simulink model "SAD_project_full_mission"  (R2023b)
settings: Solver=ode4  StartTime=0.0  StopTime=tf  FixedStep=t_step  RelTol=1e-3
values from neighbouring files (symbols this model uses):
  A1 = importdata("igrfSg.txt")    [SAD_project_code.m]
  A2 = importdata("igrfSh.txt")    [SAD_project_code.m]
  A_1 = area_face(1)    [SAD_project_code.m]
  A_2 = area_face(2)    [SAD_project_code.m]
  A_3 = area_face(3)    [SAD_project_code.m]
  A_4 = area_face(4)    [SAD_project_code.m]
  A_5 = area_face(5)    [SAD_project_code.m]
  A_6 = area_face(6)    [SAD_project_code.m]
  alpha = [1/1000 99/1000]    [SAD_project_code.m]
  DCM_eci_per = rotationMatrix(rad2deg(i),rad2deg(OM), rad2deg(om))    [SAD_project_code.m]
  e = 0.0011241    [SAD_project_code.m]
  FS = 50000e-9    (= 5e-05)    [SAD_project_code.m]
  H0 = [g_10 g_11 h_11]'    [SAD_project_code.m]
  h_r_0 = [0,0,0]'    [SAD_project_code.m]
  horizon_cone_limit = deg2rad(359)    [SAD_project_code.m]
  I = 5/12.*diag([Ix Iy Iz])    [SAD_project_code.m]
  i = deg2rad(97.55)    [SAD_project_code.m]
  I_inv = inv(I)    [SAD_project_code.m]
  I_RW = 3.32e-3    (= 0.00332)    [SAD_project_code.m]
  I_vector_RW = [I_RW I_RW I_RW]'    [SAD_project_code.m]
  inc_tot = sqrt(inc_lin^2 + inc_acc^2)    [SAD_project_code.m]
  InitialTrueAnomalyOfEarth = 0    [SAD_project_code.m]
  j_b = [0.001 0.005 0.001]'    [SAD_project_code.m]
  K1_point = lqr(A, B, Q, R)    [SAD_project_code.m]
  K1_slew = 0.8    [SAD_project_code.m]
  K2_point = K1_point.^2/2    [SAD_project_code.m]
  K2_slew = K1_slew.^2/2    [SAD_project_code.m]
  K_detumbling = lqr(A,B,Q,R)    [SAD_project_code.m]
  matrix_RW_config = eye(3)    [SAD_project_code.m]
  matrix_RW_config_inv = inv(matrix_RW_config)    [SAD_project_code.m]
  mu_E = astroConstants(13)    [SAD_project_code.m]
  N_1 = BODY(1,:)    [SAD_project_code.m]
  N_2 = BODY(2,:)    [SAD_project_code.m]
  N_3 = BODY(3,:)    [SAD_project_code.m]
  N_4 = BODY(4,:)    [SAD_project_code.m]
  N_5 = BODY(5,:)    [SAD_project_code.m]
  N_6 = BODY(6,:)    [SAD_project_code.m]
  n_earth = sqrt(mu_E/a^3)    [SAD_project_code.m]
  om = deg2rad(206.3209)    [SAD_project_code.m]
  OM = deg2rad(50.7464)    [SAD_project_code.m]
  p = a*(1-e^2)    [SAD_project_code.m]
  q0 = q0/norm(q0)    [SAD_project_code.m]
  r_1 = r(1,:)    [SAD_project_code.m]
  r_2 = r(2,:)    [SAD_project_code.m]
  r_3 = r(3,:)    [SAD_project_code.m]
  r_4 = r(4,:)    [SAD_project_code.m]
  r_5 = r(5,:)    [SAD_project_code.m]
  r_6 = r(6,:)    [SAD_project_code.m]
  R_E = astroConstants(23)    [SAD_project_code.m]
  rho_d1 = 0.1    [SAD_project_code.m]
  rho_d2 = 0.1    [SAD_project_code.m]
  rho_d3 = 0.1    [SAD_project_code.m]
  rho_d4 = 0.1    [SAD_project_code.m]
  rho_d5 = 0.1    [SAD_project_code.m]
  rho_d6 = 0.1    [SAD_project_code.m]
  rho_s1 = rho_s(1)    [SAD_project_code.m]
  rho_s2 = rho_s(2)    [SAD_project_code.m]
  rho_s3 = rho_s(3)    [SAD_project_code.m]
  rho_s4 = rho_s(4)    [SAD_project_code.m]
  rho_s5 = rho_s(5)    [SAD_project_code.m]
  rho_s6 = rho_s(6)    [SAD_project_code.m]
  t_step = 0.1    [SAD_project_code.m]
  th0 = deg2rad(0)    [SAD_project_code.m]
  timeoflaunch = date2mjd2000(date0)    [SAD_project_code.m]
  torque_max = 47.1e-3    (= 0.0471)    [SAD_project_code.m]
  ts_sensor = 5*t_step    (= 0.05)    [SAD_project_code.m]
  w0 = rand(3,1)    [SAD_project_code.m]
  w0_RW = [0 0 0]    [SAD_project_code.m]
  w_E = deg2rad(15.04)/60/60    [SAD_project_code.m]
  wMax_RW = 2*pi * RPM_max_RW / 60    (= 680.678408278)    [SAD_project_code.m]
libraries: matrix_library x28, sharedtransform x5, simulink_extras x4, simulink x3, dspindex x3, vrlib x2, dspinverses x1, aerolibutil x1
(part 1 of 4)
settings Model: Creator=samue  LastModifiedBy=samue

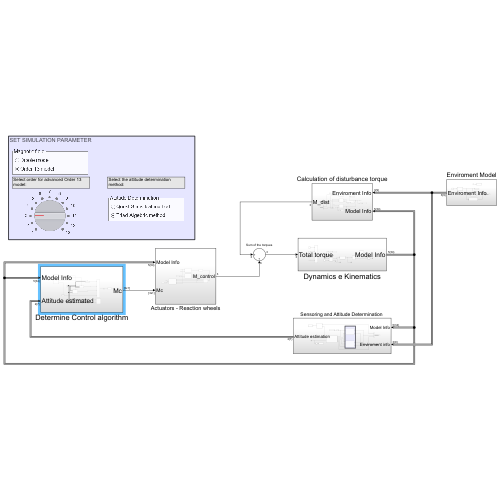
[thumbnail: Simulink's stored preview of the top-level diagram]
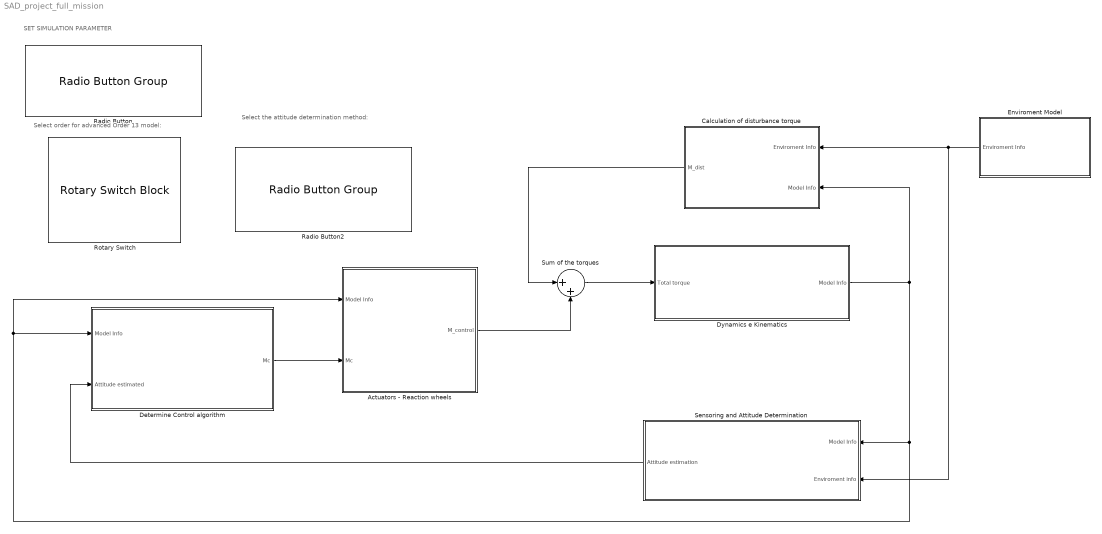
== system SAD_project_full_mission ==
  note: Select the attitude determination method:
  note: SET SIMULATION PARAMETER
  note: Select order for advanced Order 13 model:
  Actuators - Reaction wheels : Subsystem
  Calculation of disturbance torque : Subsystem
  Determine Control algorithm : Subsystem
  Dynamics e Kinematics : Subsystem
  Enviroment Model : Subsystem
  Radio Button : RadioButtonGroup  LabelPosition=Hide  SelectedLabel=Order 13 model  ButtonGroupName=Magnetic field
      settings: Values={{'Dipole model', 'Order 13 model'}, [0 1]}
  Radio Button2 : RadioButtonGroup  LabelPosition=Hide  SelectedLabel=Triad-Algebric method  ButtonGroupName=Attitude Determination
      settings: Values={{'Quest-Statisitcal method', 'Triad-Algebric method'}, [1 2]}
  Rotary Switch : RotarySwitchBlock  LabelPosition=Hide
      settings: Values={{'1', '2', '3', '4', '5', '6', '7', '8', '9', '10', '11', '12', '13'}, [1 2 3 4 5 6 7 8 9 10 11 12 13]}
  "Sensoring and Attitude Determination " : Subsystem
  Sum of the torques : Sum  Inputs=|++
  wires:
  Sum of the torques/1 -> Dynamics e Kinematics/1(Total torque)
  Actuators - Reaction wheels/1(M_control) -> Sum of the torques/2
  Enviroment Model/1(Enviroment Info) -> "Sensoring and Attitude Determination "/2(Enviroment info), Calculation of disturbance torque/1(Enviroment Info)
  Dynamics e Kinematics/1(Model Info) -> Actuators - Reaction wheels/1(Model Info), Determine Control algorithm/1(Model Info), "Sensoring and Attitude Determination "/1(Model Info), Calculation of disturbance torque/2(Model Info)
  "Sensoring and Attitude Determination "/1(Attitude estimation) -> Determine Control algorithm/2(Attitude estimated)
  Calculation of disturbance torque/1(M_dist) -> Sum of the torques/1
  Determine Control algorithm/1(Mc) -> Actuators - Reaction wheels/2(Mc)

== system SAD_project_full_mission/Actuators - Reaction wheels ==
  BusElementIn : Inport  PortName=Model Info  Element=w_b true
  Mc : Inport  Port=2
  Calculatate wRW in base of saturation : Subsystem
  Integration on omega RW : Subsystem
  Reaction wheel model : Subsystem
  Reshape : Reshape
  Reshape4 : Reshape
  Subsystem1 : Subsystem
  To Workspace1 : ToWorkspace  VariableName=wr  SampleTime=-1
  To Workspace6 : ToWorkspace  VariableName=M_actuator  SampleTime=-1
  detect if the RW is saturated (output == 1 isSaturated) : Subsystem
  M_control : Outport
  wires:
  detect if the RW is saturated (output == 1 isSaturated)/2(flag RW2) -> Calculatate wRW in base of saturation/3(flag RW2 (1 is saturated)), Subsystem1/2(flag RW2 (1 is saturated))  "flag RW2 (1 is saturated)"
  Calculatate wRW in base of saturation/1(wRW) -> Reshape/1
  Mc/1 -> Subsystem1/4(Mc), Reaction wheel model/1(Mc)
  detect if the RW is saturated (output == 1 isSaturated)/3(flag RW3) -> Calculatate wRW in base of saturation/4(flag RW3 (1 is saturated)), Subsystem1/3(flag RW3 (1 is saturated))  "flag RW3 (1 is saturated)"
  detect if the RW is saturated (output == 1 isSaturated)/1(flag RW1) -> Calculatate wRW in base of saturation/2(flag RW1 (1 is saturated)), Subsystem1/1(flag RW1 (1 is saturated))  "flag RW1 (1 is saturated)"
  Reshape/1 -> To Workspace1/1
  Subsystem1/1(M) -> M_control/1, Reshape4/1
  Reshape4/1 -> To Workspace6/1
  BusElementIn/1 -> Reaction wheel model/2(w_b true)
  Reaction wheel model/1(h_r dot) -> Integration on omega RW/1(In1)
  Integration on omega RW/1(wRW integrated) -> Calculatate wRW in base of saturation/1(wRW integrated), detect if the RW is saturated (output == 1 isSaturated)/1(w)

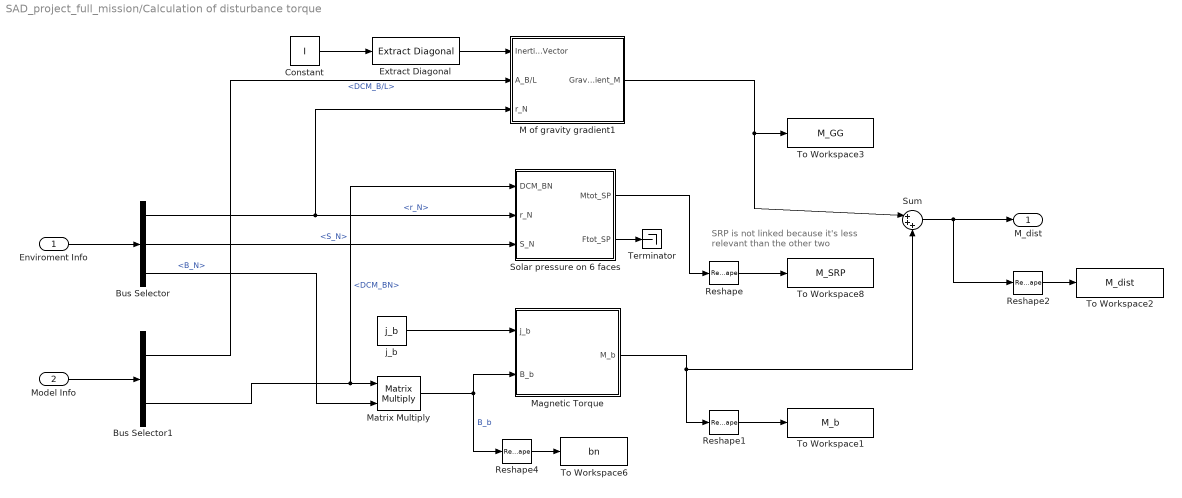
== system SAD_project_full_mission/Calculation of disturbance torque ==
  note: SRP is not linked because it's less relevant than the other two
  Enviroment Info : Inport
  Model Info : Inport  Port=2
  Bus Selector : BusSelector  OutputSignals=r_N,S_N,B_N
  Bus Selector1 : BusSelector  OutputSignals=DCM_B/L,DCM_BN
  Constant : Constant  Value=I
  Extract Diagonal : matrix_library/Extract Diagonal
      settings: LibrarySourceBlock=|
      | simulink/Matrix
      | Operations/Extract Diagonal
  M of gravity gradient1 : Subsystem
  Magnetic Torque : Subsystem
  Matrix Multiply : Product  Multiplication=Matrix(*)
  Reshape{,1..2,4} (4 alike) : Reshape
  Solar pressure on 6 faces : Subsystem
  Sum : Sum  Inputs=|+++
  Terminator : Terminator
  To Workspace1 : ToWorkspace  VariableName=M_b  SampleTime=-1
  To Workspace2 : ToWorkspace  VariableName=M_dist  SampleTime=-1
  To Workspace3 : ToWorkspace  VariableName=M_GG  SampleTime=-1
  To Workspace6 : ToWorkspace  VariableName=bn  SampleTime=-1
  To Workspace8 : ToWorkspace  VariableName=M_SRP  SampleTime=-1
  j_b : Constant  Value=j_b
  M_dist : Outport
  wires:
  j_b/1 -> Magnetic Torque/1(j_b)
  Magnetic Torque/1(M_b) -> Sum/3, Reshape1/1
  Sum/1 -> Reshape2/1, M_dist/1
  Reshape/1 -> To Workspace8/1
  Reshape1/1 -> To Workspace1/1
  M of gravity gradient1/1(GravityGradient_M) -> Sum/1, To Workspace3/1
  Solar pressure on 6 faces/2(Ftot_SP) -> Terminator/1
  Solar pressure on 6 faces/1(Mtot_SP) -> Reshape/1
  Extract Diagonal/1 -> M of gravity gradient1/1(Inertia Vector)
  Reshape4/1 -> To Workspace6/1
  Matrix Multiply/1 -> Reshape4/1, Magnetic Torque/2(B_b)  "B_b"
  Enviroment Info/1 -> Bus Selector/1
  Constant/1 -> Extract Diagonal/1
  Bus Selector/1 -> M of gravity gradient1/3(r_N), Solar pressure on 6 faces/2("r_N ")  "<r_N>"
  Bus Selector/2 -> Solar pressure on 6 faces/3(S_N)  "<S_N>"
  Model Info/1 -> Bus Selector1/1
  Bus Selector1/1 -> M of gravity gradient1/2(A_B/L)  "<DCM_B/L>"
  Reshape2/1 -> To Workspace2/1
  Bus Selector/3 -> Matrix Multiply/2  "<B_N>"
  Bus Selector1/2 -> Solar pressure on 6 faces/1(DCM_BN), Matrix Multiply/1  "<DCM_BN>"

== system SAD_project_full_mission/Determine Control algorithm ==
  Model Info : Inport
  Attitude estimated : Inport  Port=2
  Bus Selector : BusSelector  OutputSignals=q estimated
  Bus Selector1 : BusSelector  OutputSignals=A_L/N
  Check if the Mc is finite : Subsystem
  Clock : Clock
  DCM to quaternion : Subsystem
  If : If  IfExpression=u1 > 500  ElseIfExpressions=u1 > 350, u1 > 120
  Merge : Merge  Inputs=4
  "Saturation +- Max RW torque " : Saturate  UpperLimit=torque_max  LowerLimit=-torque_max
  Switch Case Action 3 axis stabilization Algorithm : Subsystem  TreatAsAtomicUnit=on
  Switch Case Action Detumle Algorithm : Subsystem  TreatAsAtomicUnit=on
  Switch Case Action Mc = 0 : Subsystem  TreatAsAtomicUnit=on
  Switch Case Action Slew Maneuver Algorithm : Subsystem  TreatAsAtomicUnit=on
  To Workspace data : Subsystem
  Mc : Outport
  wires:
  Switch Case Action Slew Maneuver Algorithm/1(Mc) -> Merge/2
  Switch Case Action Detumle Algorithm/1(Mc) -> Merge/1
  Switch Case Action 3 axis stabilization Algorithm/1(Mc) -> Merge/3
  Merge/1 -> "Saturation +- Max RW torque "/1  "Control Moment"
  Attitude estimated/1 -> Switch Case Action Slew Maneuver Algorithm/2(Attitude estimated), Switch Case Action Detumle Algorithm/1(Attitude estimated), Switch Case Action 3 axis stabilization Algorithm/2(Attitude estimated), Bus Selector/1
  Clock/1 -> If/1
  Model Info/1 -> Bus Selector1/1, Switch Case Action Slew Maneuver Algorithm/1(Model info), Switch Case Action 3 axis stabilization Algorithm/1(Model info)
  Switch Case Action Mc = 0/1(Output) -> Merge/4
  Bus Selector/1 -> To Workspace data/2(<q estimated>)  "<q estimated>"
  If/4 -> Switch Case Action Mc = 0/Action  "No control"
  If/1 -> Switch Case Action 3 axis stabilization Algorithm/Action  "3 axis Stabilisation"
  If/2 -> Switch Case Action Slew Maneuver Algorithm/Action  "Slew Maneuver"
  If/3 -> Switch Case Action Detumle Algorithm/Action  "Detumble case"
  "Saturation +- Max RW torque "/1 -> Check if the Mc is finite/1(Mc)
  Check if the Mc is finite/1(Control Moment) -> Mc/1
  Bus Selector1/1 -> DCM to quaternion/1(DCM)  "<A_L/N>"
  DCM to quaternion/1(q (scalar last)) -> To Workspace data/1(q target)

== system SAD_project_full_mission/Dynamics e Kinematics ==
  Total torque : Inport
  Constant6 : Constant  Value=q0
  DCM composition from quaternions 1 : Subsystem  AncestorBlock=LibrarySAD5/DCM composition from quaternions
  From A_B/N to A_B/L and A_L/N : Subsystem
  Inertia Matrix : Constant  Value=I  VectorParams1D=off
  "Initial ω " : Constant  Value=w0
  Inverse Inertia Matrix : Constant  Value=I_inv
  Kinematics with quaternions : Subsystem
  Matrix Multiply : Product  Multiplication=Matrix(*)
  Real Omega : ToWorkspace  VariableName=w  SampleTime=-1
  Reshape1 : Reshape
  Rotation of -90 degree around y axis : Constant  Value=[0 0 -1; 0 1 0; 1 0 0]
  Single spin dynamics : Subsystem  AncestorBlock=My_library/Single spin dynamics
  Terminator1 : Terminator
  Transpose : Math  Operator=transpose
  Out Bus Element : Outport  PortName=Model Info  Element=w_b true
  Out Bus Element2 : Outport  PortName=Model Info  Element=DCM_B/L
  Out Bus Element3 : Outport  PortName=Model Info  Element=q_b True
  Out Bus Element4 : Outport  PortName=Model Info  Element=DCM_BN
  Out Bus Element5 : Outport  PortName=Model Info  Element=A_L/N
  wires:
  Single spin dynamics/1(Omega) -> Kinematics with quaternions/1(omega), Transpose/1, Reshape1/1  "real ω_B"
  Total torque/1 -> Single spin dynamics/4(M)
  Inverse Inertia Matrix/1 -> Single spin dynamics/1(Inertia matrix inverse)
  Inertia Matrix/1 -> Single spin dynamics/2(Inertia matrix)
  "Initial ω "/1 -> Single spin dynamics/3(Omega_0)
  Constant6/1 -> Kinematics with quaternions/2(q0)
  Kinematics with quaternions/1(q) -> Out Bus Element3/1, DCM composition from quaternions 1/1(q(4x1))  "q_b True"
  Reshape1/1 -> Real Omega/1
  Kinematics with quaternions/2(q^(-1)) -> Terminator1/1
  DCM composition from quaternions 1/1(DCM) -> Out Bus Element4/1, From A_B/N to A_B/L and A_L/N/1(DCM_B/N)  "DCM_BN"
  From A_B/N to A_B/L and A_L/N/1(DCM_B/L) -> Out Bus Element2/1
  Transpose/1 -> Out Bus Element/1
  Rotation of -90 degree around y axis/1 -> Matrix Multiply/1
  From A_B/N to A_B/L and A_L/N/2(A_L/N) -> Matrix Multiply/2
  Matrix Multiply/1 -> Out Bus Element5/1

== system SAD_project_full_mission/Enviroment Model ==
  Bus Creator : BusCreator  Inputs=3
  Clock : Clock
  Constant4 : Constant  Value=th0
  Magnetic Field : Subsystem
  Sun Position in Earth Centred Equatorial Inertial RF : Subsystem
  To Workspace : ToWorkspace  VariableName=r_N  SampleTime=-1
  To Workspace1 : ToWorkspace  VariableName=t  SampleTime=-1
  two-body Keplerian dynamics ECI : Subsystem
  Enviroment Info : Outport
  wires:
  Constant4/1 -> two-body Keplerian dynamics ECI/1(th0)
  Sun Position in Earth Centred Equatorial Inertial RF/1(s_N) -> Bus Creator/2  "S_N"
  two-body Keplerian dynamics ECI/1(r_N) -> Magnetic Field/1(r_N), Bus Creator/1, To Workspace/1  "r_N"
  Magnetic Field/1(B_N) -> Bus Creator/3  "B_N"
  Bus Creator/1 -> Enviroment Info/1
  Clock/1 -> To Workspace1/1

== system SAD_project_full_mission/Sensoring and Attitude Determination  ==
  note: error between the true q and the estimated one
  note: Sensors
  Model Info : Inport
  Enviroment info : Inport  Port=2
  Attitude Determination : Subsystem
  Bus Selector : BusSelector  OutputSignals=B_N,r_N
  Bus Selector1 : BusSelector  OutputSignals=q_b True,DCM_BN,w_b true
  Horizon Sensor : Subsystem
  MAG-3  Magnetometer1 : Subsystem
  Relative attitude error with quaternion : Subsystem
  Reshape : Reshape
  Reshape3 : Reshape
  To Workspace : ToWorkspace  VariableName=w_est  SampleTime=-1
  To Workspace1 : ToWorkspace  VariableName=q_error  SampleTime=-1
  To Workspace5 : ToWorkspace  VariableName=b_sensor  SampleTime=-1
  Out Bus Element2 : Outport  PortName=Attitude estimation  Element=q estimated
  Out Bus Element1 : Outport  PortName=Attitude estimation  Element=w estimated
  wires:
  MAG-3  Magnetometer1/2(B_n) -> Attitude Determination/2(B_N)
  Horizon Sensor/1(Perturbed data Horizon) -> Attitude Determination/3(Horizon_b sensor)  "R_b perturbed sensor"
  Horizon Sensor/2(R_N Horizon) -> Attitude Determination/4(Horizon_N)
  MAG-3  Magnetometer1/1(B_b perturbed sensor) -> Attitude Determination/1(B_b sensor), Reshape3/1
  Bus Selector/1 -> MAG-3  Magnetometer1/2(B_N)  "<B_N>"
  Enviroment info/1 -> Bus Selector/1
  Bus Selector/2 -> Horizon Sensor/2(R_N)  "<r_N>"
  Bus Selector1/2 -> Horizon Sensor/1(DCM_B/N), MAG-3  Magnetometer1/1(DCM_B/N)  "<DCM_BN>"
  Reshape3/1 -> To Workspace5/1
  Model Info/1 -> Bus Selector1/1
  Relative attitude error with quaternion/1(qe) -> To Workspace1/1
  Bus Selector1/1 -> Relative attitude error with quaternion/1(q_b true)  "<q_b True>"
  Attitude Determination/1(q estimated) -> Relative attitude error with quaternion/2(estimated q), Out Bus Element2/1
  Reshape/1 -> To Workspace/1
  Attitude Determination/2(w estimated) -> Reshape/1, Out Bus Element1/1
  Horizon Sensor/3(Flag If Earth is visible) -> Attitude Determination/5(Flag IsEarthVisible)
  Bus Selector1/3 -> Attitude Determination/6(Input)  "<w_b true>"

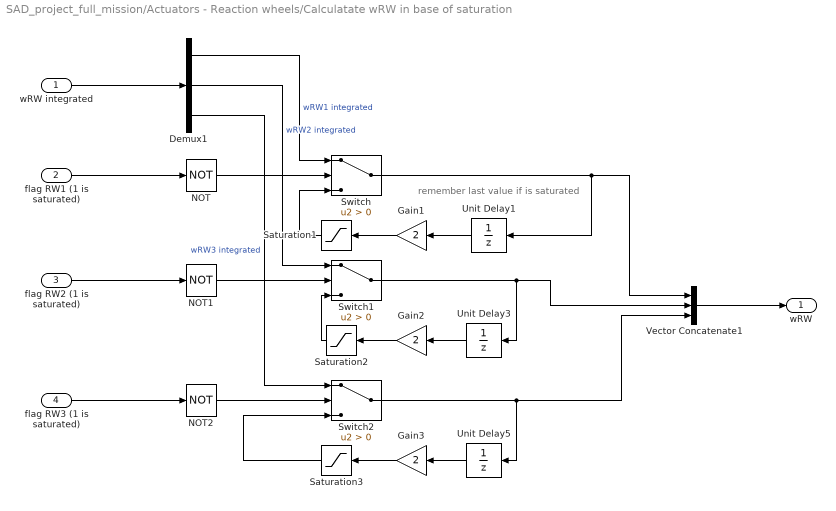
== system SAD_project_full_mission/Actuators - Reaction wheels/Calculatate wRW in base of saturation ==
  note: remember last value if is saturated
  wRW integrated : Inport
  flag RW1 (1 is saturated) : Inport  Port=2
  flag RW2 (1 is saturated) : Inport  Port=3
  flag RW3 (1 is saturated) : Inport  Port=4
  Demux1 : Demux  Outputs=3
  Gain1 : Gain  Gain=2
  Gain2 : Gain  Gain=2
  Gain3 : Gain  Gain=2
  NOT : Logic  Operator=NOT  IconShape=distinctive  AllPortsSameDT=off  OutDataTypeStr=boolean
  NOT1 : Logic  Operator=NOT  IconShape=distinctive  AllPortsSameDT=off  OutDataTypeStr=boolean
  NOT2 : Logic  Operator=NOT  IconShape=distinctive  AllPortsSameDT=off  OutDataTypeStr=boolean
  Saturation1 : Saturate  UpperLimit=wMax_RW  LowerLimit=-wMax_RW
  Saturation2 : Saturate  UpperLimit=wMax_RW  LowerLimit=-wMax_RW
  Saturation3 : Saturate  UpperLimit=wMax_RW  LowerLimit=-wMax_RW
  Switch : Switch  Criteria=u2 > Threshold  SaturateOnIntegerOverflow=off  InputSameDT=off
  Switch1 : Switch  Criteria=u2 > Threshold  SaturateOnIntegerOverflow=off  InputSameDT=off
  Switch2 : Switch  Criteria=u2 > Threshold  SaturateOnIntegerOverflow=off  InputSameDT=off
  Unit Delay1 : UnitDelay  SampleTime=-1  HasFrameUpgradeWarning=on
  Unit Delay3 : UnitDelay  SampleTime=-1  HasFrameUpgradeWarning=on
  Unit Delay5 : UnitDelay  SampleTime=-1  HasFrameUpgradeWarning=on
  Vector Concatenate1 : Concatenate  NumInputs=3
  wRW : Outport
  wires:
  Gain2/1 -> Saturation2/1
  Switch1/1 -> Unit Delay3/1, Vector Concatenate1/2
  NOT/1 -> Switch/2
  flag RW1 (1 is saturated)/1 -> NOT/1
  Saturation3/1 -> Switch2/3
  NOT1/1 -> Switch1/2
  Saturation2/1 -> Switch1/3
  wRW integrated/1 -> Demux1/1
  Switch2/1 -> Unit Delay5/1, Vector Concatenate1/3
  Unit Delay5/1 -> Gain3/1
  Unit Delay3/1 -> Gain2/1
  Demux1/2 -> Switch1/1  "wRW2 integrated"
  Gain1/1 -> Saturation1/1
  Vector Concatenate1/1 -> wRW/1
  Switch/1 -> Unit Delay1/1, Vector Concatenate1/1
  Unit Delay1/1 -> Gain1/1
  Saturation1/1 -> Switch/3
  Demux1/3 -> Switch2/1  "wRW3 integrated"
  Demux1/1 -> Switch/1  "wRW1 integrated"
  NOT2/1 -> Switch2/2
  Gain3/1 -> Saturation3/1
  flag RW3 (1 is saturated)/1 -> NOT2/1
  flag RW2 (1 is saturated)/1 -> NOT1/1

== system SAD_project_full_mission/Actuators - Reaction wheels/Integration on omega RW ==
  In1 : Inport
  Constant3 : Constant  Value=I_vector_RW
  Constant9 : Constant  Value=w0_RW
  Divide : Product  Inputs=*/
  Integrator1 : Integrator  InitialConditionSource=external
  wRW integrated : Outport
  wires:
  Divide/1 -> Integrator1/1  "wRW dot"
  Constant9/1 -> Integrator1/2
  Constant3/1 -> Divide/2
  Integrator1/1 -> wRW integrated/1  "wRW integrated"
  In1/1 -> Divide/1

== system SAD_project_full_mission/Actuators - Reaction wheels/Reaction wheel model ==
  Mc : Inport
  w_b true : Inport  Port=2
  Constant5 : Constant  Value=h_r_0  VectorParams1D=off
  Constant6 : Constant  Value=matrix_RW_config  VectorParams1D=off
  Constant8 : Constant  Value=matrix_RW_config_inv  VectorParams1D=off
  Cross Product : matrix_library/Cross Product
  Gain : Gain  Gain=-1
  Integrator : Integrator  InitialConditionSource=external
  Matrix Multiply : Product  Multiplication=Matrix(*)
  Matrix Multiply1 : Product  Multiplication=Matrix(*)
  Saturation : Saturate  UpperLimit=wMax_RW*I_RW  LowerLimit=-wMax_RW*I_RW
  Sum : Sum  Inputs=|++
  h_r dot : Outport
  wires:
  Constant5/1 -> Integrator/2
  Constant6/1 -> Matrix Multiply/1
  Sum/1 -> Matrix Multiply1/2
  Integrator/1 -> Saturation/1  "h_r"
  Matrix Multiply/1 -> Cross Product/2
  Constant8/1 -> Gain/1
  Cross Product/1 -> Sum/2
  Gain/1 -> Matrix Multiply1/1
  Matrix Multiply1/1 -> h_r dot/1, Integrator/1  "h_r dot"
  Saturation/1 -> Matrix Multiply/2
  Mc/1 -> Sum/1
  w_b true/1 -> Cross Product/1

== system SAD_project_full_mission/Actuators - Reaction wheels/Subsystem1 ==
  flag RW1 (1 is saturated) : Inport
  flag RW2 (1 is saturated) : Inport  Port=2
  flag RW3 (1 is saturated) : Inport  Port=3
  Mc : Inport  Port=4
  Band-Limited White Noise : simulink/Sources/Band-Limited White Noise  Cov=[0.00001, 0.00001, 0.00001]'  Ts=t_step  seed=[23341]
  Constant10 : Constant  Value=0
  Constant11 : Constant  Value=0
  Constant7 : Constant  Value=0
  Demux3 : Demux  Outputs=3
  Sum : Sum  Inputs=|++
  Switch1 : Switch  Criteria=u2 > Threshold  SaturateOnIntegerOverflow=off  InputSameDT=off
  Switch2 : Switch  Criteria=u2 > Threshold  SaturateOnIntegerOverflow=off  InputSameDT=off
  Switch3 : Switch  Criteria=u2 > Threshold  SaturateOnIntegerOverflow=off  InputSameDT=off
  Vector Concatenate2 : Concatenate  NumInputs=3
  M : Outport
  wires:
  Demux3/2 -> Switch1/3
  Constant11/1 -> Switch2/1
  Constant7/1 -> Switch3/1
  flag RW2 (1 is saturated)/1 -> Switch1/2
  flag RW1 (1 is saturated)/1 -> Switch3/2
  Demux3/3 -> Switch2/3
  Constant10/1 -> Switch1/1
  Demux3/1 -> Switch3/3
  flag RW3 (1 is saturated)/1 -> Switch2/2
  Switch3/1 -> Vector Concatenate2/1
  Switch1/1 -> Vector Concatenate2/2
  Switch2/1 -> Vector Concatenate2/3
  Vector Concatenate2/1 -> M/1
  Mc/1 -> Sum/1
  Sum/1 -> Demux3/1

== system SAD_project_full_mission/Actuators - Reaction wheels/detect if the RW is saturated (output == 1 isSaturated) ==
  w : Inport
  Abs : Abs  SaturateOnIntegerOverflow=off
  Compare To Constant : simulink/Logic and Bit Operations/Compare To Constant  relop=>=  const=wMax_RW  OutDataTypeStr=boolean
  Demux : Demux  Outputs=3
  Logical Operator : Logic  Operator=OR  AllPortsSameDT=off  OutDataTypeStr=boolean
  Logical Operator1 : Logic  Operator=OR  AllPortsSameDT=off  OutDataTypeStr=boolean
  Logical Operator2 : Logic  Operator=OR  AllPortsSameDT=off  OutDataTypeStr=boolean
  Unit Delay : UnitDelay  SampleTime=-1  HasFrameUpgradeWarning=on
  Unit Delay2 : UnitDelay  SampleTime=-1  HasFrameUpgradeWarning=on
  Unit Delay4 : UnitDelay  SampleTime=-1  HasFrameUpgradeWarning=on
  flag RW1 : Outport
  flag RW2 : Outport  Port=2
  flag RW3 : Outport  Port=3
  wires:
  Unit Delay4/1 -> Logical Operator2/2
  Unit Delay/1 -> Logical Operator/2
  Demux/1 -> Logical Operator/1
  Logical Operator/1 -> flag RW1/1, Unit Delay/1
  Unit Delay2/1 -> Logical Operator1/2
  Logical Operator2/1 -> flag RW3/1, Unit Delay4/1
  Demux/2 -> Logical Operator1/1
  Logical Operator1/1 -> flag RW2/1, Unit Delay2/1
  Demux/3 -> Logical Operator2/1
  Abs/1 -> Compare To Constant/1
  w/1 -> Abs/1
  Compare To Constant/1 -> Demux/1

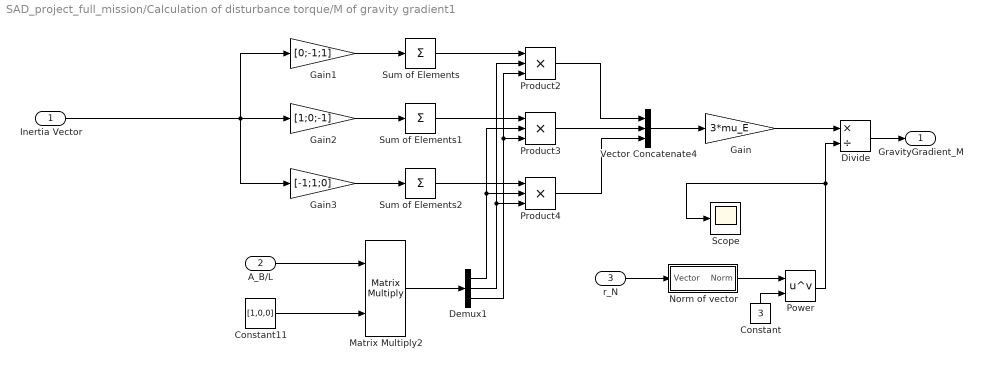
== system SAD_project_full_mission/Calculation of disturbance torque/M of gravity gradient1 ==
  Inertia Vector : Inport
  A_B/L : Inport  Port=2
  r_N : Inport  Port=3
  Constant : Constant  Value=3
  Constant11 : Constant  Value=[1,0,0]
  Demux1 : Demux  Outputs=3
  Divide : Product  Inputs=*/
  Gain : Gain  Gain=3*mu_E
  Gain1 : Gain  Gain=[0;-1;1]
  Gain2 : Gain  Gain=[1;0;-1]
  Gain3 : Gain  Gain=[-1;1;0]
  Matrix Multiply2 : Product  Multiplication=Matrix(*)
  Norm of vector : Subsystem  AncestorBlock=LibrarySAD5/Normalize Vector1
  Power : Math  Operator=pow
  Product2 : Product  Inputs=3
  Product3 : Product  Inputs=3
  Product4 : Product  Inputs=3
  Scope : Scope
  Sum of Elements : Sum  Inputs=+
  Sum of Elements1 : Sum  Inputs=+
  Sum of Elements2 : Sum  Inputs=+
  Vector Concatenate4 : Concatenate  NumInputs=3
  GravityGradient_M : Outport
  wires:
  Demux1/3 -> Product2/3, Product3/3
  Product2/1 -> Vector Concatenate4/1
  Matrix Multiply2/1 -> Demux1/1
  Product4/1 -> Vector Concatenate4/3
  Product3/1 -> Vector Concatenate4/2
  Demux1/1 -> Product4/2, Product3/2
  Constant11/1 -> Matrix Multiply2/2
  Demux1/2 -> Product4/3, Product2/2
  A_B/L/1 -> Matrix Multiply2/1
  Vector Concatenate4/1 -> Gain/1
  Gain1/1 -> Sum of Elements/1
  Gain2/1 -> Sum of Elements1/1
  Gain3/1 -> Sum of Elements2/1
  Sum of Elements/1 -> Product2/1
  Sum of Elements1/1 -> Product3/1
  Sum of Elements2/1 -> Product4/1
  Inertia Vector/1 -> Gain1/1, Gain2/1, Gain3/1
  Gain/1 -> Divide/1
  Power/1 -> Scope/1, Divide/2
  Constant/1 -> Power/2
  r_N/1 -> Norm of vector/1(Vector)
  Divide/1 -> GravityGradient_M/1
  Norm of vector/1(Norm) -> Power/1

== system SAD_project_full_mission/Calculation of disturbance torque/Magnetic Torque ==
  j_b : Inport
  B_b : Inport  Port=2
  Cross Product : matrix_library/Cross Product
  M_b : Outport
  wires:
  Cross Product/1 -> M_b/1
  j_b/1 -> Cross Product/1
  B_b/1 -> Cross Product/2

== system SAD_project_full_mission/Calculation of disturbance torque/Solar pressure on 6 faces ==
  DCM_BN : Inport
  "r_N " : Inport  Port=2
  S_N : Inport  Port=3
  Acos : Trigonometry  Operator=acos
  Dot Product : DotProduct  OutDataTypeStr=Inherit: Inherit via internal rule
  MatrixMultiply : Product  Multiplication=Matrix(*)
  MatrixMultiply1 : Product  Multiplication=Matrix(*)
  Norm of vector : Subsystem  AncestorBlock=LibrarySAD5/Normalize Vector1
  Normalize Vector : vrlib/Utilities/Normalize Vector  maxzero=0
  Normalize Vector1 : vrlib/Utilities/Normalize Vector  maxzero=0
  Solar pressure on 6 faces1 : Subsystem
  Sum1 : Sum  Inputs=|+-
  Mtot_SP : Outport
  Ftot_SP : Outport  Port=2
  wires:
  DCM_BN/1 -> MatrixMultiply1/1, MatrixMultiply/1
  S_N/1 -> Norm of vector/1(Vector), Sum1/1, MatrixMultiply/2, Normalize Vector1/1
  "r_N "/1 -> Sum1/2, MatrixMultiply1/2
  MatrixMultiply1/1 -> Solar pressure on 6 faces1/2(r_B)
  Norm of vector/1(Norm) -> Solar pressure on 6 faces1/5(s_N norm)
  MatrixMultiply/1 -> Solar pressure on 6 faces1/1(s_B)
  Sum1/1 -> Solar pressure on 6 faces1/4(S_N - r_N), Normalize Vector/1
  Normalize Vector/1 -> Dot Product/1
  Normalize Vector1/1 -> Dot Product/2
  Solar pressure on 6 faces1/1(Ftot_SP) -> Ftot_SP/1
  Dot Product/1 -> Acos/1
  Acos/1 -> Solar pressure on 6 faces1/3(S/E_S/sc_angle)
  Solar pressure on 6 faces1/2(Mtot_SP) -> Mtot_SP/1

== system SAD_project_full_mission/Determine Control algorithm/Check if the Mc is finite ==
  Mc : Inport
  Constant : Constant  Value=[0,0,0]'
  IsNaN : RelationalOperator  Operator=isNaN  OutDataTypeStr=boolean  RndMeth=Simplest  InputSameDT=off
  Norm vector : Subsystem  AncestorBlock=LibrarySAD5/Normalize Vector1
  Switch : Switch  Criteria=u2 > Threshold  SaturateOnIntegerOverflow=off  InputSameDT=off
  Control Moment : Outport
  wires:
  Constant/1 -> Switch/1
  IsNaN/1 -> Norm vector/1(Vector)
  Norm vector/1(Norm) -> Switch/2
  Mc/1 -> Switch/3, IsNaN/1
  Switch/1 -> Control Moment/1

== system SAD_project_full_mission/Determine Control algorithm/DCM to quaternion ==
  DCM : Inport
  Demux : Demux
  Direction Cosine Matrix to Quaternions1 : sharedtransform/Direction Cosine Matrix  to Quaternions  aMode=0  action=None  tolerance=eps(2)
      settings: LibrarySourceBlock=|
      | aerolibtransform2/Direction Cosine Matrix
      | to Quaternions
  Guarantee quaternion sign continuity : MATLAB Function  TreatAsAtomicUnit=on
  Mux : Mux  Inputs=3
  Unit Delay : UnitDelay  InitialCondition=q0  SampleTime=-1  HasFrameUpgradeWarning=on
  Vector Concatenate2 : Concatenate
  q (scalar last) : Outport
  wires:
  Direction Cosine Matrix to Quaternions1/1 -> Demux/1
  Demux/2 -> Mux/1
  Demux/3 -> Mux/2
  Demux/4 -> Mux/3
  Demux/1 -> Vector Concatenate2/2
  Mux/1 -> Vector Concatenate2/1
  Vector Concatenate2/1 -> Guarantee quaternion sign continuity/1("quat ")
  Unit Delay/1 -> Guarantee quaternion sign continuity/2(quat_last)
  Guarantee quaternion sign continuity/1(quat) -> q (scalar last)/1, Unit Delay/1
  DCM/1 -> Direction Cosine Matrix to Quaternions1/1

== system SAD_project_full_mission/Determine Control algorithm/Switch Case Action 3 axis stabilization Algorithm ==
  note: Linearize equation. qe is the error between q target e q current
      | K1 is definite using LQR function. K2 is define using K2 = sqrt(2*k1)
      | Saturation block to limit Control torque
  BusElementIn : Inport  PortName=Model info  Element=A_L/N
  BusElementIn2 : Inport  Port=2  PortName=Attitude estimated  Element=q estimated
  BusElementIn3 : Inport  Port=2  PortName=Attitude estimated  Element=w estimated
  Action Port : ActionPort  PropagateVarSize=During execution  ActionPortLabel=if(u1 > 500)
  Constant : Constant  Value=[0,0,n_earth]'
  Constant1 : Constant  Value=-K2_point
  Constant2 : Constant  Value=K1_point
  DCM to quaternion1 : Subsystem
  Demux1 : Demux
  Gain : Gain  Gain=2
  Matrix Multiply1 : Product  Multiplication=Matrix(*)
  Matrix Multiply2 : Product  Multiplication=Matrix(*)
  Product2 : Product
  Relative attitude error quaternion3 : Subsystem
  Sum : Sum  Inputs=|-+
  Sum1 : Sum  Inputs=|+-
  Vector Concatenate1 : Concatenate  NumInputs=3
  Mc : Outport
  wires:
  BusElementIn2/1 -> Relative attitude error quaternion3/2(q2 (Estimated))
  Relative attitude error quaternion3/1(qe) -> Demux1/1
  Matrix Multiply1/1 -> Gain/1
  DCM to quaternion1/1(q (scalar last)1) -> Relative attitude error quaternion3/1(q1 (usually Target))
  Demux1/2 -> Vector Concatenate1/2
  Demux1/3 -> Vector Concatenate1/3
  Constant2/1 -> Matrix Multiply2/1
  Constant1/1 -> Matrix Multiply1/1
  Vector Concatenate1/1 -> Matrix Multiply1/2
  Product2/1 -> Sum1/1
  Demux1/4 -> Product2/2
  BusElementIn3/1 -> Matrix Multiply2/2
  Demux1/1 -> Vector Concatenate1/1
  Sum1/1 -> Mc/1
  BusElementIn/1 -> DCM to quaternion1/1(DCM)
  Gain/1 -> Product2/1
  Matrix Multiply2/1 -> Sum/2
  Sum/1 -> Sum1/2
  Constant/1 -> Sum/1

== system SAD_project_full_mission/Determine Control algorithm/Switch Case Action Detumle Algorithm ==
  note: Q and R weight are choosen limiting the maximum values of states and control
      | Q = diag([1/1, 1/1, 1/1]);
      | R = diag([1/max_torque^2, 1/ max_torque^2 , 1/ max_torque^2 ]);
  Attitude estimated : Inport
  Action Port : ActionPort  PropagateVarSize=During execution  ActionPortLabel=elseif( u1 > 120)
  Bus Selector : BusSelector  OutputSignals=w estimated
  Constant : Constant  Value=K_detumbling
  Gain : Gain  Gain=-1
  Matrix Multiply : Product  Multiplication=Matrix(*)
  Scope : Scope
  Mc : Outport
  wires:
  Attitude estimated/1 -> Bus Selector/1
  Bus Selector/1 -> Scope/1, Matrix Multiply/2  "<w estimated>"
  Constant/1 -> Gain/1
  Gain/1 -> Matrix Multiply/1
  Matrix Multiply/1 -> Mc/1

== system SAD_project_full_mission/Determine Control algorithm/Switch Case Action Mc = 0 ==
  Action Port : ActionPort  PropagateVarSize=During execution  ActionPortLabel=else
  Constant : Constant  Value=[0 0 0]'
  Output : Outport
  wires:
  Constant/1 -> Output/1

== system SAD_project_full_mission/Determine Control algorithm/Switch Case Action Slew Maneuver Algorithm ==
  note: Non linear equation. Where u = Mc and \delta H(q4e) = 1 - q4e
      | K1 is definite using LQR function. K2 is define using K2 = sqrt(2*k1)
      | Saturation block to limit Control torque
  BusElementIn : Inport  PortName=Model info  Element=A_L/N
  BusElementIn4 : Inport  PortName=Model info  Element=w_b true
  BusElementIn2 : Inport  Port=2  PortName=Attitude estimated  Element=q estimated
  BusElementIn3 : Inport  Port=2  PortName=Attitude estimated  Element=w estimated
  Action Port : ActionPort  ActionPortLabel=elseif(u1 > 350)
  -(K_2*J) : Constant  Value=-(K2_slew*I)
  Constant3 : Constant  Value=I
  DCM to quaternion1 : Subsystem
  I*K_1 : Constant  Value=K1_slew*I
  Matrix Multiply : Product  Multiplication=Matrix(*)
  Matrix Multiply1 : Product  Multiplication=Matrix(*)
  Product2 : Product
  "Quaternion Decomposition " : Demux
  Relative attitude error quaternion3 : Subsystem
  Sum1 : Sum  Inputs=|++-
  Vector Concatenate1 : Concatenate  NumInputs=3
  "cross(w, Iw)" : Subsystem
  Mc : Outport
  wires:
  Relative attitude error quaternion3/1(qe) -> "Quaternion Decomposition "/1
  BusElementIn2/1 -> Relative attitude error quaternion3/2(q2 (Estimated))
  -(K_2*J)/1 -> Matrix Multiply1/1
  "Quaternion Decomposition "/4 -> Product2/2  "qe4"
  "Quaternion Decomposition "/1 -> Vector Concatenate1/1  "qe1"
  "Quaternion Decomposition "/3 -> Vector Concatenate1/3  "qe3"
  DCM to quaternion1/1(q (scalar last)1) -> Relative attitude error quaternion3/1(q1 (usually Target))
  "Quaternion Decomposition "/2 -> Vector Concatenate1/2  "qe2"
  Vector Concatenate1/1 -> Matrix Multiply1/2
  BusElementIn3/1 -> Matrix Multiply/2
  Product2/1 -> Sum1/2
  BusElementIn/1 -> DCM to quaternion1/1(DCM)  "Target"
  BusElementIn4/1 -> "cross(w, Iw)"/1(w)
  Constant3/1 -> "cross(w, Iw)"/2(Inertia)
  "cross(w, Iw)"/1("cross(w, Iw)") -> Sum1/1
  Matrix Multiply1/1 -> Product2/1
  Matrix Multiply/1 -> Sum1/3
  I*K_1/1 -> Matrix Multiply/1
  Sum1/1 -> Mc/1

== system SAD_project_full_mission/Determine Control algorithm/To Workspace data ==
  q target : Inport
  <q estimated> : Inport  Port=2
  Demux : Demux
  Error to Target in degree : ToWorkspace  VariableName=degree_target_error  SampleTime=-1
  Mux : Mux
  Output Target : ToWorkspace  VariableName=q_target  SampleTime=-1
  Output error : ToWorkspace  VariableName=q_errorTarget  SampleTime=-1
  Quaternions to Rotation Angles : sharedtransform/Quaternions to Rotation Angles  rotationOrder=ZYX  aMode=aMode
  Radians to Degrees : simulink_extras/Transformations/Radians to Degrees
  Relative attitude error quaternion target-current : Subsystem
  Reshape{,1..3} (4 alike) : Reshape
  To Workspace : ToWorkspace  VariableName=q_est  SampleTime=-1
  wires:
  <q estimated>/1 -> Relative attitude error quaternion target-current/2(q2 (Estimated)), Reshape3/1
  Demux/2 -> Mux/3
  Demux/4 -> Mux/1
  Reshape3/1 -> To Workspace/1
  Relative attitude error quaternion target-current/1(qe) -> Demux/1, Reshape/1
  Quaternions to Rotation Angles/1 -> Radians to Degrees/1
  Reshape1/1 -> Error to Target in degree/1
  Radians to Degrees/1 -> Reshape1/1
  Mux/1 -> Quaternions to Rotation Angles/1
  q target/1 -> Relative attitude error quaternion target-current/1(q1 (usually Target)), Reshape2/1
  Reshape/1 -> Output error/1
  Demux/3 -> Mux/4
  Reshape2/1 -> Output Target/1
  Demux/1 -> Mux/2

== system SAD_project_full_mission/Dynamics e Kinematics/DCM composition from quaternions 1 ==
  q(4x1) : Inport
  Cross product matrix composition : Subsystem
  Demux : Demux
  Dot Product : DotProduct  OutDataTypeStr=Inherit: Inherit via internal rule
  Gain : Gain  Gain=[1 0 0; 0 1 0; 0 0 1]
  Gain1 : Gain  Gain=2
  Gain2 : Gain  Gain=-2
  Mux : Mux  Inputs=3
  Product : Product  Multiplication=Matrix(*)
  Product1 : Product
  Square : Math  Operator=square
  Sum : Sum  Inputs=|-+
  Sum1 : Sum  Inputs=+++
  Transpose : Math  Operator=transpose
  DCM : Outport
  wires:
  Gain/1 -> Sum1/1
  Demux/1 -> Mux/1
  q(4x1)/1 -> Demux/1
  Demux/2 -> Mux/2
  Mux/1 -> Dot Product/2, Dot Product/1, Product/1, Cross product matrix composition/1(q_vect), Transpose/1  "q_vect"
  Demux/4 -> Gain2/1, Square/1  "q4"
  Demux/3 -> Mux/3
  Dot Product/1 -> Sum/1
  Sum/1 -> Gain/1
  Square/1 -> Sum/2
  Transpose/1 -> Product/2
  Product/1 -> Gain1/1
  Gain2/1 -> Product1/2
  Cross product matrix composition/1(q_vect cross) -> Product1/1  "omega_mat"
  Product1/1 -> Sum1/3
  Gain1/1 -> Sum1/2
  Sum1/1 -> DCM/1

== system SAD_project_full_mission/Dynamics e Kinematics/From A_B//N to A_B//L and A_L//N ==
  DCM_B/N : Inport
  Constant : Constant  Value=th0
  Integration of true anomaly : Subsystem
  calculating A_B/L : Subsystem
  DCM_B/L : Outport
  A_L/N : Outport  Port=2
  wires:
  calculating A_B/L/1(A_B/L) -> DCM_B/L/1
  DCM_B/N/1 -> calculating A_B/L/2(A_B/N)
  calculating A_B/L/2(A_L/N) -> A_L/N/1
  Integration of true anomaly/1(th) -> calculating A_B/L/1(Theta)  "Theta"
  Constant/1 -> Integration of true anomaly/1(th0)

== system SAD_project_full_mission/Dynamics e Kinematics/Kinematics with quaternions ==
  omega : Inport
  q0 : Inport  Port=2
  Demux : Demux
  Divide : Product  Inputs=*/
  Gain1 : Gain  Gain=-1
  Gain2 : Gain  Gain=-1
  Gain3 : Gain  Gain=1/2
  Gain4 : Gain  Gain=-1
  Integrator : Integrator  InitialConditionSource=external
  Matrix Multiply : Product  Multiplication=Matrix(*)
  Matrix OMEGA : Subsystem
  Mux : Mux
  Normalize Vector2 : Subsystem
  q : Outport
  q^(-1) : Outport  Port=2
  wires:
  Gain3/1 -> Matrix Multiply/1
  Matrix Multiply/1 -> Integrator/1  "q_dot"
  omega/1 -> Matrix OMEGA/1(omega)
  Integrator/1 -> Divide/1, Normalize Vector2/1(Vector), Demux/1, q/1  "q"
  Matrix OMEGA/1(Matrix Omega) -> Gain3/1
  q0/1 -> Integrator/2
  Demux/2 -> Gain1/1
  Demux/3 -> Gain2/1
  Demux/4 -> Gain4/1
  Gain1/1 -> Mux/2
  Gain2/1 -> Mux/3
  Gain4/1 -> Mux/4
  Demux/1 -> Mux/1
  Mux/1 -> q^(-1)/1
  Normalize Vector2/1(Norm) -> Divide/2
  Divide/1 -> Matrix Multiply/2

== system SAD_project_full_mission/Dynamics e Kinematics/Single spin dynamics ==
  Inertia matrix inverse : Inport
  Inertia matrix : Inport  Port=2
  Omega_0 : Inport  Port=3
  M : Inport  Port=4
  Cross Product : matrix_library/Cross Product
  Integrator1 : Integrator  InitialConditionSource=external
  Product : Product  Multiplication=Matrix(*)
  Product1 : Product  Multiplication=Matrix(*)
  Sum : Sum  Inputs=|++
  Transpose1 : Math  Operator=transpose
  Omega : Outport
  wires:
  Transpose1/1 -> Omega/1
  Inertia matrix inverse/1 -> Product/1
  Integrator1/1 -> Product1/2, Transpose1/1, Cross Product/2  "omega"
  Product/1 -> Integrator1/1  "omega_dot"
  Omega_0/1 -> Integrator1/2
  Product1/1 -> Cross Product/1
  Inertia matrix/1 -> Product1/1
  Cross Product/1 -> Sum/1
  Sum/1 -> Product/2
  M/1 -> Sum/2

== system SAD_project_full_mission/Enviroment Model/Magnetic Field ==
  r_N : Inport
  Control by check box : Constant
  Merge : Merge
  Switch Case Action Adavanced Magnetic model : Subsystem  TreatAsAtomicUnit=on
  Switch Case Action Dipole model : Subsystem  TreatAsAtomicUnit=on
  Switch Case2 : SwitchCase
  B_N : Outport
  wires:
  Switch Case Action Dipole model/1(b_N) -> Merge/2
  Switch Case2/1 -> Switch Case Action Adavanced Magnetic model/Action
  Switch Case2/2 -> Switch Case Action Dipole model/Action
  Control by check box/1 -> Switch Case2/1
  r_N/1 -> Switch Case Action Adavanced Magnetic model/1(r_N), Switch Case Action Dipole model/1(r_N)
  Switch Case Action Adavanced Magnetic model/1(B_n) -> Merge/1
  Merge/1 -> B_N/1

== system SAD_project_full_mission/Enviroment Model/Sun Position in Earth Centred Equatorial Inertial RF ==
  note: pointing Sun from Earth
      | x=vernal line
      | y=perpendicular
      | z=cnp
  Clock : Clock
  Gain : Gain  Gain=cos(23.45/360*2*pi)
  Gain1 : Gain  Gain=sin(23.45/360*2*pi)
  InitialTrueAnomalyOfEarth : Constant  Value=InitialTrueAnomalyOfEarth
  MatrixMultiply : Product
  Mux : Mux  Inputs=3
  Product : Product
  Sum : Sum  Inputs=|++
  Trigonometric Function : Trigonometry  Operator=cos
  Trigonometric Function1 : Trigonometry
  mean ang vel : Constant  Value=2*pi/31536000
  mean distance : Constant  Value=149597870
  s_N : Outport
  wires:
  Trigonometric Function/1 -> Mux/1
  Gain1/1 -> Mux/3
  Mux/1 -> MatrixMultiply/2
  MatrixMultiply/1 -> s_N/1  "s_N"
  mean distance/1 -> MatrixMultiply/1
  Gain/1 -> Mux/2
  Trigonometric Function1/1 -> Gain1/1, Gain/1
  mean ang vel/1 -> Product/2
  Clock/1 -> Product/1
  InitialTrueAnomalyOfEarth/1 -> Sum/2
  Product/1 -> Sum/1
  Sum/1 -> Trigonometric Function1/1, Trigonometric Function/1

== system SAD_project_full_mission/Enviroment Model/two-body Keplerian dynamics ECI ==
  th0 : Inport
  Constant : Constant  Value=DCM_eci_per
  Integration of true anomaly : Subsystem
  Matrix Multiply : Product  Multiplication=Matrix(*)
  Transpose : Math  Operator=transpose
  r_perifocal : Subsystem
  r_N : Outport
  wires:
  th0/1 -> Integration of true anomaly/1(th0)
  Integration of true anomaly/1(th) -> r_perifocal/1(th)
  Constant/1 -> Transpose/1
  Transpose/1 -> Matrix Multiply/1
  r_perifocal/1(r_per) -> Matrix Multiply/2
  Matrix Multiply/1 -> r_N/1

== system SAD_project_full_mission/Sensoring and Attitude Determination /Attitude Determination ==
  note: If flag==0, the case selected switches to case 3 -> only magnetometer
  B_b sensor : Inport
  B_N : Inport  Port=2
  Horizon_b sensor : Inport  Port=3
  Horizon_N : Inport  Port=4
  Flag IsEarthVisible : Inport  Port=5
  Input : Inport  Port=6
  Constant1 : Constant  Value=2
  From q to omega : Subsystem
  If Action Subsystem : Subsystem  TreatAsAtomicUnit=on
  If Action Subsystem1 : Subsystem  TreatAsAtomicUnit=on
  If1 : If  IfExpression="u1  == 3"
  Merge : Merge  Inputs=3
  Merge1 : Merge
  Switch Case : SwitchCase  CaseConditions={1,2,3}  ShowDefaultCase=off
  Switch Case Action Only-Magnetometer : Subsystem  TreatAsAtomicUnit=on
  Switch Case Action Statisitcal Attitude : Subsystem  TreatAsAtomicUnit=on
  Switch Case Action Triad Case : Subsystem  TreatAsAtomicUnit=on
  q estimated : Outport
  w estimated : Outport  Port=2
  wires:
  Merge/1 -> q estimated/1, From q to omega/1(q estimated)  "q estimated"
  B_N/1 -> Switch Case Action Only-Magnetometer/2(B_N), Switch Case Action Triad Case/3(B_N), Switch Case Action Statisitcal Attitude/3(B_N)
  From q to omega/1(estimated w) -> w estimated/1
  Switch Case Action Statisitcal Attitude/1(Out1) -> Merge/1
  Switch Case Action Triad Case/1(Output) -> Merge/2
  B_b sensor/1 -> Switch Case Action Only-Magnetometer/1(B_b sensor), Switch Case Action Triad Case/1(B_b sensor), Switch Case Action Statisitcal Attitude/1(B_b sensor)
  Horizon_b sensor/1 -> Switch Case Action Triad Case/2(Horizon_b sensor), Switch Case Action Statisitcal Attitude/2(Horizon_b sensor)
  Horizon_N/1 -> Switch Case Action Triad Case/4(Horizon_N), Switch Case Action Statisitcal Attitude/4(Horizon_N)
  Switch Case/1 -> Switch Case Action Statisitcal Attitude/Action  "QUEST"
  Switch Case/2 -> Switch Case Action Triad Case/Action  "TRIAD"
  If Action Subsystem1/1(3) -> Merge1/1
  If1/2 -> If Action Subsystem/Action
  Flag IsEarthVisible/1 -> If Action Subsystem/2(Flag horizon)
  Constant1/1 -> If Action Subsystem/1(Attitude method choice), If1/1
  If1/1 -> If Action Subsystem1/Action
  If Action Subsystem/1(method) -> Merge1/2
  Merge1/1 -> Switch Case/1
  Switch Case/3 -> Switch Case Action Only-Magnetometer/Action
  Input/1 -> Switch Case Action Only-Magnetometer/3(w_true)
  Switch Case Action Only-Magnetometer/1(q (scalar last)) -> Merge/3

== system SAD_project_full_mission/Sensoring and Attitude Determination /Horizon Sensor ==
  DCM_B/N : Inport
  R_N : Inport  Port=2
  Add noise of 1 deg : simulink/Sources/Band-Limited White Noise  Cov=[0.00001 0.00001 0]  Ts=ts_sensor  seed=[23341]
  Constant : Constant  Value=horizon_cone_limit
  From s/c to Earth : Gain  Gain=-1
  Normalize Vector : Subsystem
  Rotation in body frame : Product  Multiplication=Matrix(*)
  Rotation in body frame1 : Product  Multiplication=Matrix(*)
  Sum : Sum  Inputs=|++
  Switch : Switch  Criteria=u2 > Threshold  SaturateOnIntegerOverflow=off  InputSameDT=off
  True Roll and Pitch betwen nadir and -z_body1 : Subsystem
  Unit Delay : UnitDelay  InitialCondition=[0 1 0]'  SampleTime=-1  HasFrameUpgradeWarning=on
  Zero-Order Hold : ZeroOrderHold  SampleTime=ts_sensor
  perturbed -R_B when Horizon does not see the Earth : Constant  Value=[1 1 1]
  Perturbed data Horizon : Outport
  R_N Horizon : Outport  Port=2
  Flag If Earth is visible : Outport  Port=3
  wires:
  Zero-Order Hold/1 -> Rotation in body frame1/2
  True Roll and Pitch betwen nadir and -z_body1/1(Flag if sensor sees Earth) -> Switch/2, Flag If Earth is visible/1
  Normalize Vector/1(Versor) -> Rotation in body frame/2
  Rotation in body frame1/1 -> Sum/1
  DCM_B/N/1 -> Rotation in body frame1/1, Rotation in body frame/1
  Switch/1 -> Unit Delay/1
  Add noise of 1 deg/1 -> Sum/2
  Sum/1 -> Switch/1
  perturbed -R_B when Horizon does not see the Earth/1 -> Switch/3
  R_N/1 -> From s/c to Earth/1  "R_N Sat Earth vector"
  From s/c to Earth/1 -> Zero-Order Hold/1, Normalize Vector/1(Vector), R_N Horizon/1
  Unit Delay/1 -> Perturbed data Horizon/1
  Rotation in body frame/1 -> True Roll and Pitch betwen nadir and -z_body1/1(R_b)  "R_b unperturbed body frame"
  Constant/1 -> True Roll and Pitch betwen nadir and -z_body1/2(cone_limit_angle)

== system SAD_project_full_mission/Sensoring and Attitude Determination /MAG-3  Magnetometer1 ==
  note: CODE TO ADD TO MAKE SENSOR WORK
      | % Time definition
      | t0 = 0;
      | tf = T; %Period of orbit
      | t_step = 0.01; %fixed step of simulation
      | ts_sensor = t_step; % Sample of sensor (can change but must to be a multiple of t_step)
      |
      | % MAG-3 sensor data and error
      | FS = 500e-9; %Full scale value
      | inc_lin = 0.15/100; % Accuracy error
      | inc_acc = 0.75/100; % Linear error
      | inc_tot = sqrt(inc_lin^2 + inc_acc^2); %Total error
  DCM_B/N : Inport
  B_N : Inport  Port=2
  Error gain of sensor MAG-3 : Gain  Gain=inc_tot*FS
  Rotation in body frame : Product  Multiplication=Matrix(*)
  Saturation to FS : Saturate  UpperLimit=FS  LowerLimit=-FS
  Sum : Sum  Inputs=|++
  Unit Delay : UnitDelay  InitialCondition=[0,0,1]'  SampleTime=-1  HasFrameUpgradeWarning=on
  Vector Concatenate : Concatenate  NumInputs=3
  White Noise : RandomNumber  DisableCoverage=on  Seed=1  SampleTime=ts_sensor
  White Noise1 : RandomNumber  DisableCoverage=on  Seed=2  SampleTime=ts_sensor
  White Noise2 : RandomNumber  DisableCoverage=on  Seed=3  SampleTime=ts_sensor
  Zero-Order Hold : ZeroOrderHold  SampleTime=ts_sensor
  B_b perturbed sensor : Outport
  B_n : Outport  Port=2
  wires:
  Vector Concatenate/1 -> Error gain of sensor MAG-3/1
  White Noise/1 -> Vector Concatenate/1
  Error gain of sensor MAG-3/1 -> Sum/2
  White Noise2/1 -> Vector Concatenate/3
  White Noise1/1 -> Vector Concatenate/2
  DCM_B/N/1 -> Rotation in body frame/1
  B_N/1 -> B_n/1, Zero-Order Hold/1
  Saturation to FS/1 -> Unit Delay/1
  Rotation in body frame/1 -> Sum/1
  Sum/1 -> Saturation to FS/1
  Zero-Order Hold/1 -> Rotation in body frame/2
  Unit Delay/1 -> B_b perturbed sensor/1

== system SAD_project_full_mission/Sensoring and Attitude Determination /Relative attitude error with quaternion ==
  q_b true : Inport
  estimated q : Inport  Port=2
  Demux : Demux
  Gain1 : Gain  Gain=[0,0,0,-1; 0,0,1,0; 0,-1,0 0; 1,0,0,0]
  Gain2 : Gain  Gain=[0, 0, -1 ,0; 0, 0 ,0 ,-1; 1, 0, 0, 0; 0 1, 0, 0]
  Gain3 : Gain  Gain=[0 1 0 0; -1 0 0 0; 0 0 0 -1; 0 0 1 0]
  Gain4 : Gain  Gain=eye(4)
  Matrix Multiply : Product  Multiplication=Matrix(*)
  Sum1 : Sum  Inputs=++++
  qe : Outport
  wires:
  Gain1/1 -> Sum1/1
  Demux/2 -> Gain2/1
  Gain3/1 -> Sum1/3
  Demux/1 -> Gain1/1
  Sum1/1 -> Matrix Multiply/1
  Demux/3 -> Gain3/1
  Gain4/1 -> Sum1/4
  Gain2/1 -> Sum1/2
  Demux/4 -> Gain4/1
  estimated q/1 -> Matrix Multiply/2
  Matrix Multiply/1 -> qe/1
  q_b true/1 -> Demux/1

== system SAD_project_full_mission/Calculation of disturbance torque/M of gravity gradient1/Norm of vector ==
  Vector : Inport
  Dot Product : DotProduct  OutDataTypeStr=Inherit: Inherit via internal rule
  Sqrt : Sqrt
  Norm : Outport
  wires:
  Sqrt/1 -> Norm/1
  Vector/1 -> Dot Product/1, Dot Product/2
  Dot Product/1 -> Sqrt/1

== system SAD_project_full_mission/Calculation of disturbance torque/Solar pressure on 6 faces/Norm of vector ==
  Vector : Inport
  Dot Product : DotProduct  OutDataTypeStr=Inherit: Inherit via internal rule
  Sqrt : Sqrt
  Norm : Outport
  wires:
  Sqrt/1 -> Norm/1
  Vector/1 -> Dot Product/1, Dot Product/2
  Dot Product/1 -> Sqrt/1
